simulink model "DebugScreen"  (R2018a)
settings: Solver=FixedStepAuto  StartTime=0.0  StopTime=40  FixedStep=0.05  RelTol=1e-3
undefined symbols (not defined in the file): CR, serial
libraries: instrumentlib x5, uartLib x1
settings Model: Creator=SIMONE  LastModifiedBy=SIMONE

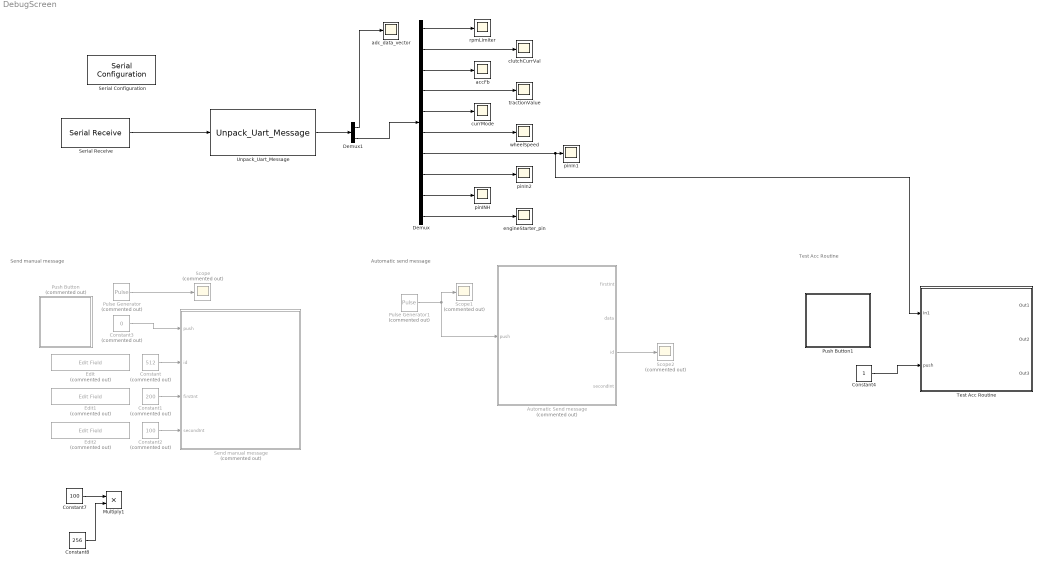
== system DebugScreen ==
  note: Test Acc Routine
  note: Automatic send message
  note: Send manual message
  Automatic Send message : Stateflow chart  Commented=on  TreatAsAtomicUnit=on
  Constant : Constant  Commented=on  Value=512  OutDataTypeStr=uint16
  Constant1 : Constant  Commented=on  Value=200  OutDataTypeStr=uint16
  Constant2 : Constant  Commented=on  Value=100  OutDataTypeStr=uint16
  Constant3 : Constant  Commented=on  Value=0
  Constant4 : Constant
  Constant7 : Constant  Value=100  OutDataTypeStr=uint16
  Constant8 : Constant  Value=256  OutDataTypeStr=uint16
  Demux : Demux  Outputs=10
  Demux1 : Demux  Outputs=2
  Edit : EditField  Commented=on  WebBlockId=20  LabelPosition=Hide  Alignment=Center
  Edit1 : EditField  Commented=on  WebBlockId=23  LabelPosition=Hide  Alignment=Center
  Edit2 : EditField  Commented=on  WebBlockId=25  LabelPosition=Hide  Alignment=Center
  Multiply1 : Product  OutDataTypeStr=uint16
  Pulse Generator : DiscretePulseGenerator  Commented=on  PulseType=Time based  Period=10  PulseWidth=2%  PhaseDelay=1
  Pulse Generator1 : DiscretePulseGenerator  Commented=on  PulseType=Time based  Period=0.2  PulseWidth=25%  PhaseDelay=1
  Push Button : Subsystem  Commented=on  DialogController=hmiCreateDDGDialog  IsWebBlock=on  mask(MWDashboardBlock){webBlockId=12b47424-de0c-4dac-be92-db9266863398, webBlockType=pushbutton, ShowInLibBrwoser=on, ShowInitialText=on, HMISrcModelName=DebugScreen}
      mask prompts: webBlockId "WebBlock Id"; webBlockType "WebBlock Type"; HMISrcModelName "Source Model"
      mask help: SimulinkHMI:dialogs:PushButtonDialogDesc
      mask Help: helpview([docroot '/mapfiles/simulink.map'], 'hmi_push_button')
      mask Display:
      | model = bdroot(gcb);
      | if strcmp(get_param(model,'BlockDiagramType'), 'library')
      |     image([(matlabroot) '/toolbox/simulink/hmi/icons/PushButton.png']);
      | end
  Push Button1 : Subsystem  DialogController=hmiCreateDDGDialog  IsWebBlock=on  mask(MWDashboardBlock){webBlockId=b87c9129-2ae4-4d53-baa3-891c0a6e6068, webBlockType=pushbutton, ShowInLibBrwoser=on, ShowInitialText=on, HMISrcModelName=DebugScreen}
      mask prompts: webBlockId "WebBlock Id"; webBlockType "WebBlock Type"; HMISrcModelName "Source Model"
      mask help: SimulinkHMI:dialogs:PushButtonDialogDesc
      mask Help: helpview([docroot '/mapfiles/simulink.map'], 'hmi_push_button')
      mask Display:
      | model = bdroot(gcb);
      | if strcmp(get_param(model,'BlockDiagramType'), 'library')
      |     image([(matlabroot) '/toolbox/simulink/hmi/icons/PushButton.png']);
      | end
  Scope : Scope  Commented=on
  Scope1 : Scope  Commented=on
  Scope2 : Scope  Commented=on
  Send manual message : Stateflow chart  Commented=on  TreatAsAtomicUnit=on
  Serial Configuration : instrumentlib/Serial Configuration  Priority=-200000  ComPortMenu=COM4  ComPort=COM4  ObjConstructor=serial('COM4');  BaudRate=115200  DataBits=8  Parity=none  StopBits=1  FlowControl=none  Timeout=10  ByteOrder=LittleEndian
  Serial Receive : instrumentlib/Serial Receive  ComPortMenu=COM4  ComPort=COM4  ObjConstructor=serial('COM4');  Header=hdr  Terminator=CR ('\r')  DataSize="[40   1]"  DataType=uint8  EnableBlockingMode=on  ActionDataUnavailable=Output last received value  CustomValue=0  SampleTime=0.05
  Test Acc Routine : Subsystem
  Unpack_Uart_Message : uartLib/Unpack_Uart_Message  SFunctionModules=''
  accFb : Scope
  adc_data_vector : Scope
  clutchCurrVal : Scope
  currMode : Scope
  engineStarter_pin : Scope
  pinINH : Scope
  pinIn1 : Scope
  pinIn2 : Scope
  rpmLimiter : Scope
  tractionValue : Scope
  wheelSpeed : Scope
  wires:
  Serial Receive/1 -> Unpack_Uart_Message/1
  Demux/7 -> Test Acc Routine/1(In1), pinIn1/1
  Constant2/1 -> Send manual message/4(secondInt)
  Constant/1 -> Send manual message/2(id)
  Pulse Generator/1 -> Scope/1
  Pulse Generator1/1 -> Scope1/1, Automatic Send message/1(push)
  Automatic Send message/3(id) -> Scope2/1
  Demux/3 -> accFb/1
  Demux/1 -> rpmLimiter/1
  Demux/8 -> pinIn2/1
  Constant3/1 -> Send manual message/1(push)
  Constant4/1 -> Test Acc Routine/2(push)
  Constant7/1 -> Multiply1/1
  Constant8/1 -> Multiply1/2
  Constant1/1 -> Send manual message/3(firstInt)
  Unpack_Uart_Message/1 -> Demux1/1
  Demux1/1 -> adc_data_vector/1
  Demux1/2 -> Demux/1
  Demux/2 -> clutchCurrVal/1
  Demux/4 -> tractionValue/1
  Demux/6 -> wheelSpeed/1
  Demux/5 -> currMode/1
  Demux/9 -> pinINH/1
  Demux/10 -> engineStarter_pin/1

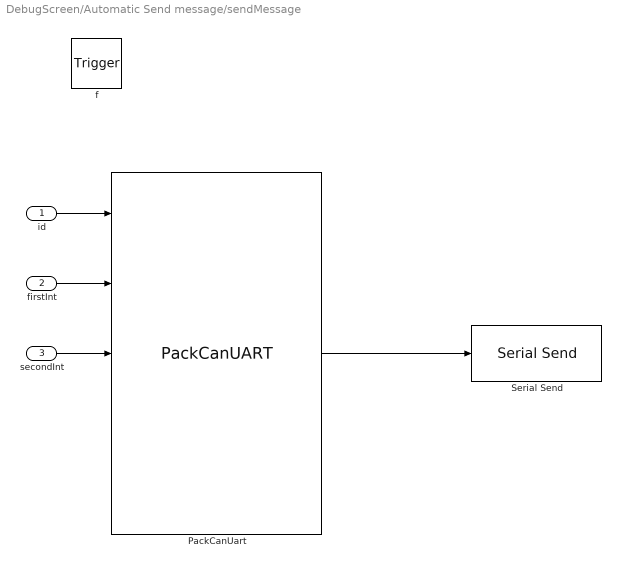
== system DebugScreen/Automatic Send message/sendMessage ==
  id : Inport  OutDataTypeStr=uint16  PortDimensions=1
  firstInt : Inport  Port=2  OutDataTypeStr=uint16  PortDimensions=1
  secondInt : Inport  Port=3  OutDataTypeStr=uint16  PortDimensions=1
  f : TriggerPort  TriggerType=function-call  VariantControl=(inherit)
      settings: CopyFcn=Stateflow.SLINSF.SimulinkMan.removeBlockPreDeleteFcn  PreDeleteFcn=Stateflow.SLINSF.SimulinkMan.unsafePredeleteFcn
  PackCanUart : S-Function  FunctionName=PackCanUART  SFunctionDeploymentMode=off  EnableBusSupport=off
  Serial Send : instrumentlib/Serial Send  ComPortMenu=<Please select a port...>  ComPort=COM4  ObjConstructor=serial('COM4');  Header=hdr  Terminator=<none>  EnableBlockingMode=on
  wires:
  secondInt/1 -> PackCanUart/3
  firstInt/1 -> PackCanUart/2
  PackCanUart/1 -> Serial Send/1
  id/1 -> PackCanUart/1

== system DebugScreen/Push Button ==

== system DebugScreen/Push Button1 ==

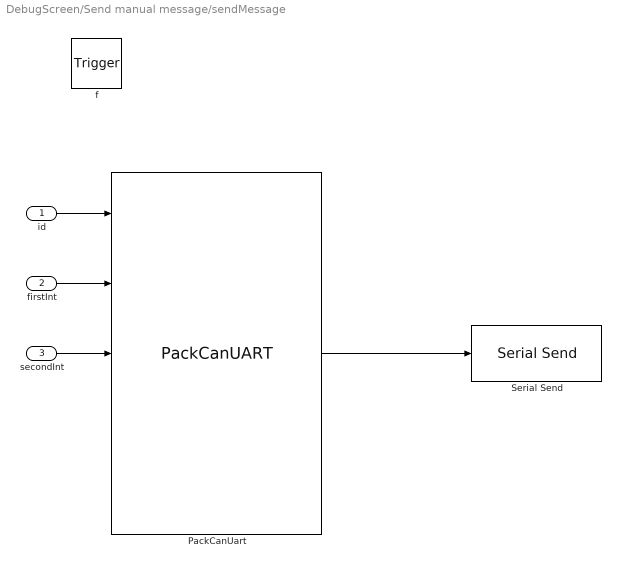
== system DebugScreen/Send manual message/sendMessage ==
  id : Inport  OutDataTypeStr=uint16  PortDimensions=1
  firstInt : Inport  Port=2  OutDataTypeStr=uint16  PortDimensions=1
  secondInt : Inport  Port=3  OutDataTypeStr=uint16  PortDimensions=1
  f : TriggerPort  TriggerType=function-call  VariantControl=(inherit)
      settings: CopyFcn=Stateflow.SLINSF.SimulinkMan.removeBlockPreDeleteFcn  PreDeleteFcn=Stateflow.SLINSF.SimulinkMan.unsafePredeleteFcn
  PackCanUart : S-Function  FunctionName=PackCanUART  SFunctionDeploymentMode=off  EnableBusSupport=off
  Serial Send : instrumentlib/Serial Send  ComPortMenu=COM4  ComPort=COM4  ObjConstructor=serial('COM4');  Header=hdr  Terminator=<none>  EnableBlockingMode=on
  wires:
  secondInt/1 -> PackCanUart/3
  firstInt/1 -> PackCanUart/2
  PackCanUart/1 -> Serial Send/1
  id/1 -> PackCanUart/1

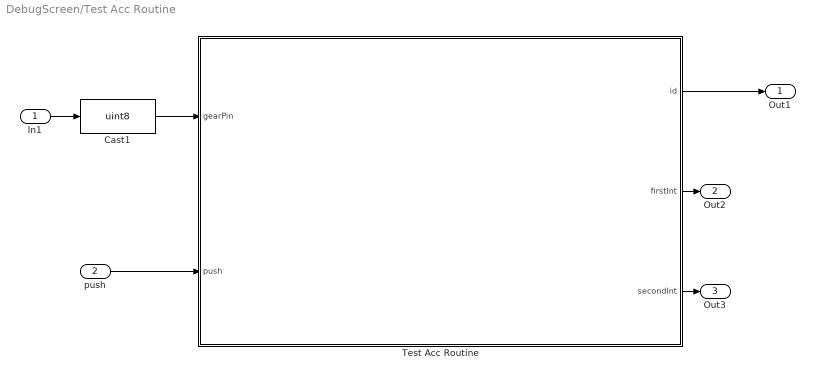
== system DebugScreen/Test Acc Routine ==
  In1 : Inport
  push : Inport  Port=2
  Cast1 : DataTypeConversion  OutDataTypeStr=uint8
  Test Acc Routine : Stateflow chart  TreatAsAtomicUnit=on  SystemSampleTime=0.05
  Out1 : Outport
  Out2 : Outport  Port=2
  Out3 : Outport  Port=3
  wires:
  In1/1 -> Cast1/1
  Test Acc Routine/1(id) -> Out1/1
  Cast1/1 -> Test Acc Routine/1(gearPin)
  Test Acc Routine/3(secondInt) -> Out3/1
  Test Acc Routine/2(firstInt) -> Out2/1
  push/1 -> Test Acc Routine/2(push)

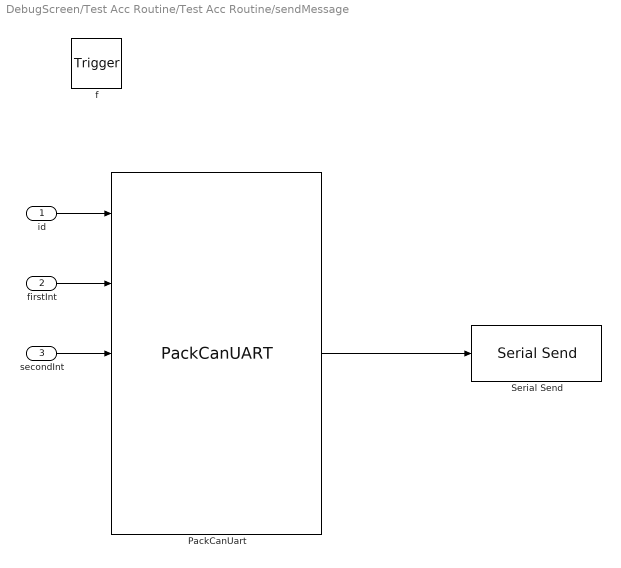
== system DebugScreen/Test Acc Routine/Test Acc Routine/sendMessage ==
  id : Inport  OutDataTypeStr=uint16  PortDimensions=1
  firstInt : Inport  Port=2  OutDataTypeStr=uint16  PortDimensions=1
  secondInt : Inport  Port=3  OutDataTypeStr=uint16  PortDimensions=1
  f : TriggerPort  TriggerType=function-call  VariantControl=(inherit)
      settings: CopyFcn=Stateflow.SLINSF.SimulinkMan.removeBlockPreDeleteFcn  PreDeleteFcn=Stateflow.SLINSF.SimulinkMan.unsafePredeleteFcn
  PackCanUart : S-Function  FunctionName=PackCanUART  SFunctionDeploymentMode=off  EnableBusSupport=off
  Serial Send : instrumentlib/Serial Send  ComPortMenu=<Please select a port...>  ComPort=COM4  ObjConstructor=serial('COM12');  Header=hdr  Terminator=<none>  EnableBlockingMode=on
  wires:
  secondInt/1 -> PackCanUart/3
  firstInt/1 -> PackCanUart/2
  PackCanUart/1 -> Serial Send/1
  id/1 -> PackCanUart/1

== stateflow chart DebugScreen/Send manual message ==
  state sendMessage(id,firstInt,secondInt) [function]
  state No_push
  state Push
    entry:
    sendMessage(id, firstInt, secondInt);
  (default) -> No_push
  No_push -> Push : [push==1]
  Push -> No_push : [push==0]
  data: id function_input uint16 size=1; firstInt function_input uint16 size=1; secondInt function_input uint16 size=1; push input; id input uint16; firstInt input uint16; secondInt input uint16

== stateflow chart DebugScreen/Automatic Send message ==
  state sendMessage(id,firstInt,secondInt) [function]
  state Add [commented out]
    entry:
    %firstInt = 512;
    firstInt=firstInt+256
    sendMessage(id, firstInt, secondInt);
    data = firstInt/256;
  state Subtract [commented out]
    entry:
    %firstInt = 1024;
    firstInt=firstInt+256
    sendMessage(id, firstInt, secondInt);
    data = firstInt/256;
  state setClutch
    entry:
    id = 513;
    firstInt = 65535;
    sendMessage(id, firstInt, secondInt);
  state aacCom
    entry:
    id = 514;
    firstInt = 1;
    sendMessage(id, firstInt, secondInt);
  state GearUpdate
    entry:
    id = 773;
    firstInt=1;
    secondInt = 1000;
    sendMessage(id, firstInt, secondInt);
  state ChangeGear
    entry:
    id = 512;
    firstInt = 400;
    sendMessage(id, firstInt, secondInt);
  state changeMode
    entry:
    id = 1000;
    firstInt = 3;
    sendMessage(id, firstInt, secondInt);
  state aacCom1
    entry:
    id = 514;
    firstInt = 0;
    sendMessage(id, firstInt, secondInt);
  (default) -> Add [commented out]
  Add -> Subtract [commented out] : [data<100]
  Subtract -> Add [commented out] : [data<100]
  (default) -> GearUpdate
  GearUpdate -> setClutch : [push ==1]
  setClutch -> aacCom : [push ==1]
  aacCom -> changeMode : [push ==1]
  changeMode -> aacCom1 : [push ==1]
  aacCom1 -> ChangeGear : [push ==1]
  data: id function_input uint16 size=1; firstInt function_input uint16 size=1; secondInt function_input uint16 size=1; push input; firstInt output uint16 =uint16(0); data output uint16 =uint16(0); id output uint16 =uint16(0); secondInt output uint16 =uint16(0)

== stateflow chart DebugScreen/Test Acc Routine/Test Acc Routine ==
  state Routine [parallel]
    settings: executionOrder=1
    state Wait
    state updateData [function]
      (default) -> (junction 20)
      (junction 20) -> (junction 24) [order 1] : [gearPin == 0 && lastGearPin == 1]
      (junction 20) -> (junction 22) [order 2]
      (junction 24) -> (junction 26) : { currGear = currGear + 1;}
      (junction 26) -> (junction 39)
      (junction 39) -> (junction 43)
      (junction 22) -> (junction 28) [order 1] : [gearPin == 1]
      (junction 22) -> (junction 30) [order 2] : {rpm = rpm + 150; wheelSpeed = wheelSpeed + 5;}
      (junction 28) -> (junction 33) : {rpm = 0; wheelSpeed = 0;}
      (junction 30) -> (junction 33) [order 1] : [message == 0]
      (junction 30) -> (junction 37) [order 2] : {message = 0; id = 774; firstInt = wheelSpeed;}
      (junction 33) -> (junction 35) : {message =1; id = 773; firstInt = currGear; secondInt = rpm;}
      (junction 37) -> (junction 35)
      (junction 35) -> (junction 43)
      (junction 43) -> (junction 46) : {lastGearPin = gearPin;}
    state InsertGear
      entry:
      id = uint16(512);
      firstInt = uint16(400);
      sendMessage(id,firstInt,secondInt)
      during:
      checkGear;
    state Ready
      id = uint16(514);
      firstInt = uint16(2);
      sendMessage(id,firstInt,secondInt)
    state EnterAcceleration
      id = uint16(1000);
      firstInt = uint16(3);
      sendMessage(id,firstInt,secondInt)
    state ActivateAac
      entry:
      id = uint16(514);
      firstInt = uint16(1);
      sendMessage(id,firstInt,secondInt)
    state DajeDeGas
      entry:
      id = uint16(0);
      rpm = uint16(0);
      wheelSpeed = uint16(0);
      during:
      updateData;
      sendMessage(id,firstInt,secondInt)
    state checkGear [function]
      (default) -> (junction 55)
      (junction 55) -> (junction 57) [order 1] : [gearPin == 0 && lastGearPin ==1]
      (junction 55) -> (junction 61) [order 2]
      (junction 57) -> (junction 59) : {currGear = currGear + 1;}
      (junction 59) -> (junction 64)
      (junction 61) -> (junction 64)
      (junction 64) -> (junction 67) : {lastGearPin = gearPin}
    state EXIT
      entry:
      id = uint16(513);
      firstInt = bitshift(uint16(100), 8);
    (default) -> Wait
    Wait -> EnterAcceleration : [push==1]
    InsertGear -> Ready : [currGear ==1 && push==1]
    EnterAcceleration -> ActivateAac : [push==1]
    ActivateAac -> InsertGear : [push==1]
    Ready -> DajeDeGas
    DajeDeGas -> EXIT [commented out] : [currGear==5]
  state sendMessage(id,firstInt,secondInt) [function]
  data: id function_input uint16 size=1; firstInt function_input uint16 size=1; secondInt function_input uint16 size=1; id output uint16 =uint16(0); firstInt output uint16 =uint16(0); secondInt output uint16 =uint16(0);; counter local; gearPin input uint8; lastGearPin local uint8 =uint8(0); message local =0; rpm local uint16; wheelSpeed local uint16; currGear local uint16 =uint16(0);; count local; push input
